simulink model "act3_simulink_sesion2"  (R2020a)
settings: Solver=ode1  StartTime=0.0  StopTime=30  FixedStep=0.5  RelTol=1e-3
settings Model: Creator=Jorjolo  LastModifiedBy=Jorjolo

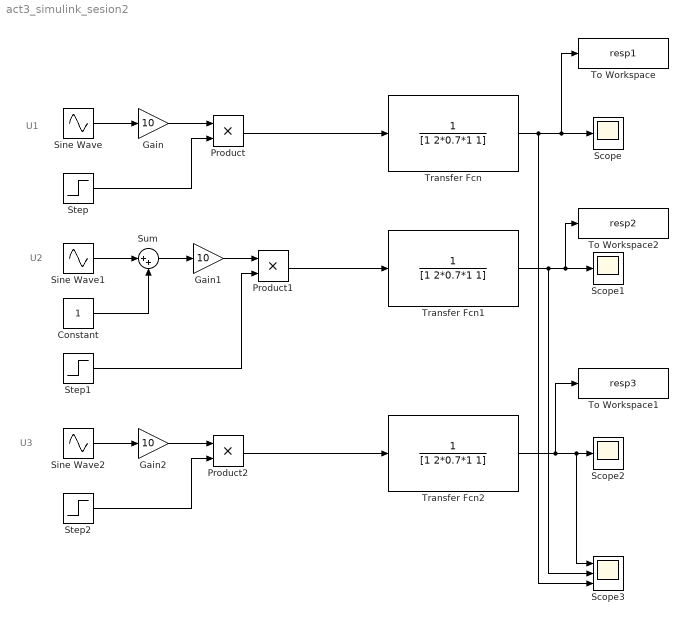
== system act3_simulink_sesion2 ==
  note: U3
  note: U2
  note: U1
  Constant : Constant
  Gain : Gain  Gain=10
  Gain1 : Gain  Gain=10
  Gain2 : Gain  Gain=10
  Product : Product
  Product1 : Product
  Product2 : Product
  Scope : Scope
  Scope1 : Scope
  Scope2 : Scope
  Scope3 : Scope  NumInputPorts=3
  Sine Wave : Sin  Frequency=3  SampleTime=0
  Sine Wave1 : Sin  Frequency=3  SampleTime=0
  Sine Wave2 : Sin  Frequency=10  SampleTime=0
  Step : Step  Time=0  SampleTime=0
  Step1 : Step  Time=0  SampleTime=0
  Step2 : Step  Time=0  SampleTime=0
  Sum : Sum  Inputs=|++
  To Workspace : ToWorkspace  VariableName=resp1  SaveFormat=Timeseries  SampleTime=-1
  To Workspace1 : ToWorkspace  VariableName=resp3  SaveFormat=Timeseries  SampleTime=-1
  To Workspace2 : ToWorkspace  VariableName=resp2  SaveFormat=Timeseries  SampleTime=-1
  Transfer Fcn : TransferFcn  Numerator=[0 1]  Denominator=[1 2*0.7*1 1]
  Transfer Fcn1 : TransferFcn  Numerator=[0 1]  Denominator=[1 2*0.7*1 1]
  Transfer Fcn2 : TransferFcn  Numerator=[0 1]  Denominator=[1 2*0.7*1 1]
  wires:
  Sine Wave/1 -> Gain/1
  Gain/1 -> Product/1
  Step/1 -> Product/2
  Gain2/1 -> Product2/1
  Sine Wave2/1 -> Gain2/1
  Step2/1 -> Product2/2
  Sine Wave1/1 -> Sum/1
  Constant/1 -> Sum/2
  Sum/1 -> Gain1/1
  Gain1/1 -> Product1/1
  Step1/1 -> Product1/2
  Product/1 -> Transfer Fcn/1
  Product1/1 -> Transfer Fcn1/1
  Product2/1 -> Transfer Fcn2/1
  Transfer Fcn/1 -> Scope3/3, To Workspace/1, Scope/1
  Transfer Fcn1/1 -> Scope3/2, To Workspace2/1, Scope1/1
  Transfer Fcn2/1 -> To Workspace1/1, Scope3/1, Scope2/1
